simulink model "ACC"  (R2018a)
settings: Solver=VariableStepAuto  StartTime=0.0  StopTime=10.0  RelTol=1e-3
settings Model: Creator=Manchey  LastModifiedBy=Manchey

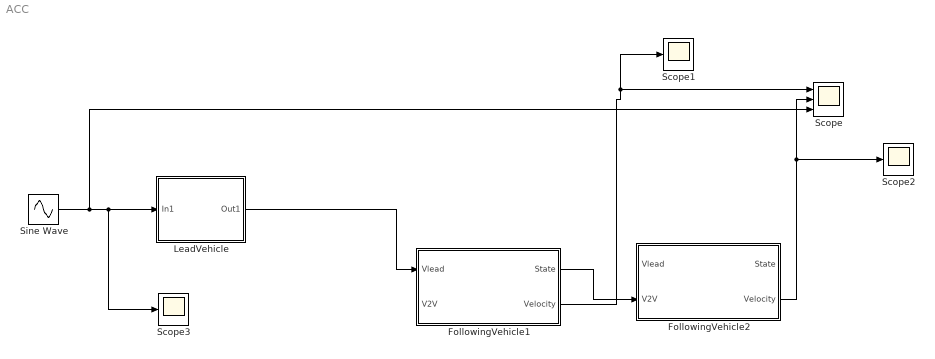
== system ACC ==
  FollowingVehicle1 : Subsystem
  FollowingVehicle2 : Subsystem
  LeadVehicle : Subsystem
  Scope : Scope  NumInputPorts=3
  Scope1 : Scope
  Scope2 : Scope
  Scope3 : Scope
  Sine Wave : Sin  Amplitude=12  SampleTime=0
  wires:
  LeadVehicle/1(Out1) -> FollowingVehicle1/1(Vlead)
  Sine Wave/1 -> Scope/3, Scope3/1, LeadVehicle/1(In1)
  FollowingVehicle1/1(State) -> FollowingVehicle2/2(V2V)
  FollowingVehicle1/2(Velocity) -> Scope1/1, Scope/1
  FollowingVehicle2/2(Velocity) -> Scope2/1, Scope/2

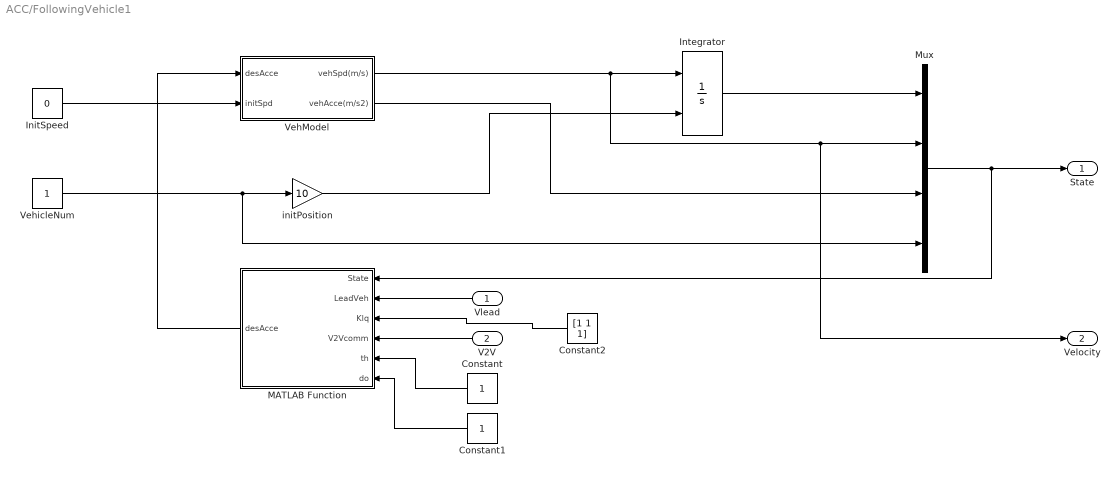
== system ACC/FollowingVehicle1 ==
  Vlead : Inport
  V2V : Inport  Port=2
  Constant : Constant
  Constant1 : Constant
  Constant2 : Constant  Value=[1 1 1]
  InitSpeed : Constant  Value=0
  Integrator : Integrator  InitialConditionSource=external
  MATLAB Function : MATLAB Function  TreatAsAtomicUnit=on
  Mux : Mux
  VehModel : Subsystem
  VehicleNum : Constant
  initPosition : Gain  Gain=10
  State : Outport
  Velocity : Outport  Port=2
  wires:
  Vlead/1 -> MATLAB Function/2(LeadVeh)
  initPosition/1 -> Integrator/2
  Constant/1 -> MATLAB Function/5(th)
  MATLAB Function/1(desAcce) -> VehModel/1(desAcce)
  Constant2/1 -> MATLAB Function/3(Klq)
  VehModel/2(vehAcce(m/s2)) -> Mux/3
  Mux/1 -> State/1, MATLAB Function/1(State)
  Constant1/1 -> MATLAB Function/6(do)
  Integrator/1 -> Mux/1
  InitSpeed/1 -> VehModel/2(initSpd)
  VehicleNum/1 -> Mux/4, initPosition/1
  V2V/1 -> MATLAB Function/4(V2Vcomm)
  VehModel/1(vehSpd(m/s)) -> Velocity/1, Mux/2, Integrator/1

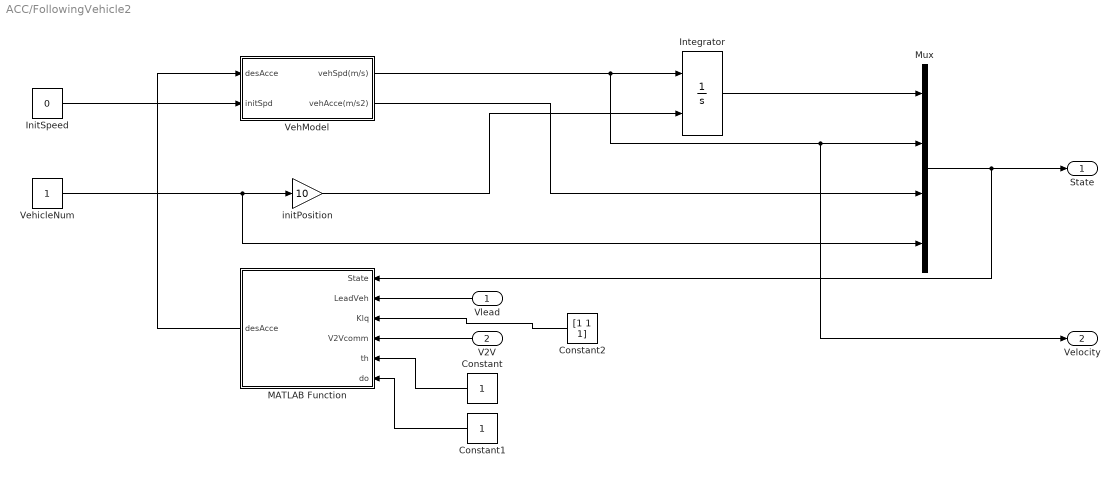
== system ACC/FollowingVehicle2 ==
  Vlead : Inport
  V2V : Inport  Port=2
  Constant : Constant
  Constant1 : Constant
  Constant2 : Constant  Value=[1 1 1]
  InitSpeed : Constant  Value=0
  Integrator : Integrator  InitialConditionSource=external
  MATLAB Function : MATLAB Function  TreatAsAtomicUnit=on
  Mux : Mux
  VehModel : Subsystem
  VehicleNum : Constant
  initPosition : Gain  Gain=10
  State : Outport
  Velocity : Outport  Port=2
  wires:
  Vlead/1 -> MATLAB Function/2(LeadVeh)
  initPosition/1 -> Integrator/2
  Constant/1 -> MATLAB Function/5(th)
  MATLAB Function/1(desAcce) -> VehModel/1(desAcce)
  Constant2/1 -> MATLAB Function/3(Klq)
  VehModel/2(vehAcce(m/s2)) -> Mux/3
  Mux/1 -> State/1, MATLAB Function/1(State)
  Constant1/1 -> MATLAB Function/6(do)
  Integrator/1 -> Mux/1
  InitSpeed/1 -> VehModel/2(initSpd)
  VehicleNum/1 -> Mux/4, initPosition/1
  V2V/1 -> MATLAB Function/4(V2Vcomm)
  VehModel/1(vehSpd(m/s)) -> Velocity/1, Mux/2, Integrator/1

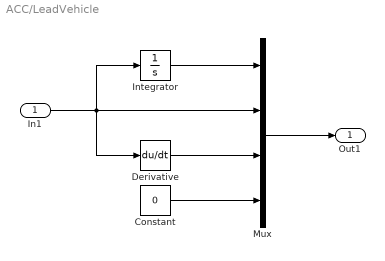
== system ACC/LeadVehicle ==
  In1 : Inport
  Constant : Constant  Value=0
  Derivative : Derivative
  Integrator : Integrator
  Mux : Mux
  Out1 : Outport
  wires:
  Mux/1 -> Out1/1
  Integrator/1 -> Mux/1
  In1/1 -> Derivative/1, Mux/2, Integrator/1
  Derivative/1 -> Mux/3
  Constant/1 -> Mux/4

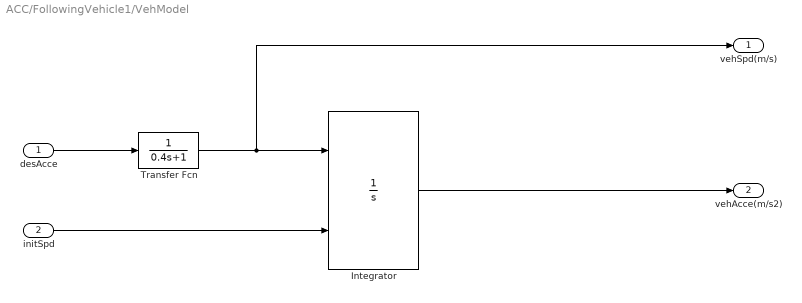
== system ACC/FollowingVehicle1/VehModel ==
  desAcce : Inport
  initSpd : Inport  Port=2
  Integrator : Integrator  InitialConditionSource=external  LimitOutput=on  UpperSaturationLimit=100  LowerSaturationLimit=0
  Transfer Fcn : TransferFcn  Denominator=[0.4 1]
  vehSpd(m/s) : Outport
  vehAcce(m/s2) : Outport  Port=2
  wires:
  desAcce/1 -> Transfer Fcn/1
  Transfer Fcn/1 -> vehSpd(m/s)/1, Integrator/1
  initSpd/1 -> Integrator/2
  Integrator/1 -> vehAcce(m/s2)/1

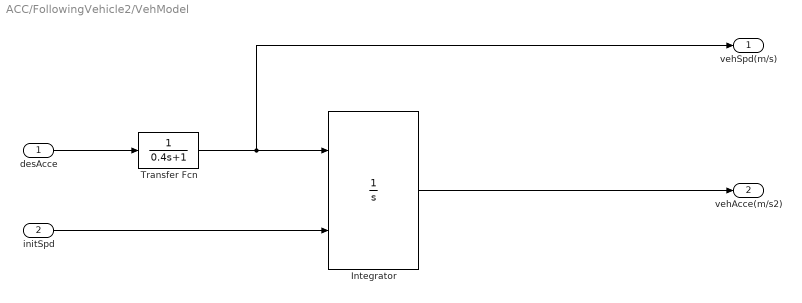
== system ACC/FollowingVehicle2/VehModel ==
  desAcce : Inport
  initSpd : Inport  Port=2
  Integrator : Integrator  InitialConditionSource=external  LimitOutput=on  UpperSaturationLimit=100  LowerSaturationLimit=0
  Transfer Fcn : TransferFcn  Denominator=[0.4 1]
  vehSpd(m/s) : Outport
  vehAcce(m/s2) : Outport  Port=2
  wires:
  desAcce/1 -> Transfer Fcn/1
  Transfer Fcn/1 -> vehSpd(m/s)/1, Integrator/1
  initSpd/1 -> Integrator/2
  Integrator/1 -> vehAcce(m/s2)/1

== matlab function ACC/FollowingVehicle2/MATLAB Function ==
  data: State input; desAcce output; LeadVeh input; Klq input; V2Vcomm input; th input; do input
function desAcce = fcn(State, LeadVeh, Klq, V2Vcomm, th, do)
%% Initial Parameters
VehNum = State(4);

%% Control Input from Lead Vehicle
CtrlLead = 0;
if length(LeadVeh) == 1
    CtrlLead(1) = 0;
    Lveh = 0;
else
    Lveh = LeadVeh(2);
    desDist = th*Lveh+do;
    CtrlLead(1) = (Klq(1)*(LeadVeh(1)-State(1)-VehNum*desDist)...
                    +Klq(2)*(LeadVeh(2)-State(2))...
                    +Klq(3)*(LeadVeh(3)-State(3)));
end

%% Control Input from V2V
n_states_Follow = length(V2Vcomm);
if n_states_Follow == 1
    ctrinputs=0;
else
    n_sgns = n_states_Follow/4;
    ctrinputs=zeros(1,n_sgns);

    for i = 1:n_sgns
        desDist = th*State(2) + do;
        ctrinputs(i) = (Klq(1)*(V2Vcomm(1+(i-1)*4)-State(1)-(VehNum-V2Vcomm(i*4))*desDist)...
                    +Klq(2)*(V2Vcomm(2+(i-1)*4)-State(2))...
                    +Klq(3)*(V2Vcomm(3+(i-1)*4)-State(3)));
    end
end

%% Sum of control signals
desAcce = sum(ctrinputs) + CtrlLead(1);

== matlab function ACC/FollowingVehicle1/MATLAB Function ==
  data: State input; desAcce output; LeadVeh input; Klq input; V2Vcomm input; th input; do input
function desAcce = fcn(State, LeadVeh, Klq, V2Vcomm, th, do)
%% Initial Parameters
VehNum = State(4);

%% Control Input from Lead Vehicle
CtrlLead = 0;
if length(LeadVeh) == 1
    CtrlLead(1) = 0;
    Lveh = 0;
else
    Lveh = LeadVeh(2);
    desDist = th*Lveh+do;
    CtrlLead(1) = (Klq(1)*(LeadVeh(1)-State(1)-VehNum*desDist)...
                    +Klq(2)*(LeadVeh(2)-State(2))...
                    +Klq(3)*(LeadVeh(3)-State(3)));
end

%% Control Input from V2V
n_states_Follow = length(V2Vcomm);
if n_states_Follow == 1
    ctrinputs=0;
else
    n_sgns = n_states_Follow/4;
    ctrinputs=zeros(1,n_sgns);
    for i = 1:n_sgns
        desDist = th*State(2) + do;
        ctrinputs(i) = (Klq(1)*(V2Vcomm(1+(i-1)*4)-State(1)-(VehNum-V2Vcomm(i*4))*desDist)...
                    +Klq(2)*(V2Vcomm(2+(i-1)*4)-State(2))...
                    +Klq(3)*(V2Vcomm(3+(i-1)*4)-State(3)));
    end
end

%% Sum of control signals
desAcce = sum(ctrinputs) + CtrlLead(1);
